simulink model "vdc_dyc_v3"  (R2020a)
settings: Solver=ode4  StartTime=0.0  StopTime=inf  FixedStep=1e-3  RelTol=1e-3
InitFcn:
  | clear mex
values from neighbouring files (symbols this model uses):
  vicrt_inputfile = append(path_send,              '2261_VOLCANO_ramp_RH12002_send_svm.xml')    [select_maneuver_files.m]
undefined symbols (not defined in the file or in its folder): vicrt_initcallback, vicrt_initmexcallback, vicrt_simulationmanager
libraries: simulink x1
(part 2 of 5)

== system vdc_dyc_v3/2261 VOLCANO PL7 MY22 R03/VI-CarRealTime/Input_Bus/Bus2Map ==
  Bus In : Inport
  Bus Selector : BusSelector  OutputSignals=Driver_Demands.str_swa,Subsystem_Activation.Internal_Steering_Column_Activity,Driver_Demands.rack_displacement,Driver_Demands.throttle,Driver_Demands.gear,Driver_Demands.clutch,Driver_Demands.brake,Driver_Demands.target_speed,Driver_Demands.target_acc,Brake_System_General.brk_mast_cyl_pres,Brake_System_General.brk_bias_front,ABS.Internal_ABS_Activity,ABS.ABS_threshold,Driver_Demands.user_maneuver_ID,Driver_Demands.user_input_steering,Driver_Demands.user_input_throttle,Driver_Demands.user_input_braking,Driver_Demands.user_input_gear,Driver_Demands.user_input_clutch,TCS.Internal_TCS_Activity,TCS.TCS_threshold,Friction.tire_mu.L1,Friction.tire_mu.L2,Friction.tire_mu.R1,Friction.tire_mu.R2,Subsystem_Activation.Internal_Brake_System_Activity.L1,Brake_System.brk_mmag_sign.L1,Brake_System.brk_mmag_unsign.L1,Brake_System.brk_pres.L1,Brake_System.brk_pres_gain.L1,Brake_System.brk_mu.L1,Subsystem_Activation.Internal_Brake_System_Activity.L2,Brake_System.brk_mmag_sign.L2,Brake_System.brk_mmag_unsign.L2,Brake_System.brk_pres.L2,Brake_System.brk_pres_gain.L2,Brake_System.brk_mu.L2,Subsystem_Activation.Internal_Brake_System_Activity.R1,Brake_System.brk_mmag_sign.R1,Brake_System.brk_mmag_unsign.R1,Brake_System.brk_pres.R1,Brake_System.brk_pres_gain.R1,Brake_System.brk_mu.R1,Subsystem_Activation.Internal_Brake_System_Activity.R2,Brake_System.brk_mmag_sign.R2,Brake_System.brk_mmag_unsign.R2,Brake_System.brk_pres.R2,Brake_System.brk_pres_gain.R2,Brake_System.brk_mu.R2,Hook.Fx.rear,Hook.Fy.rear,Hook.Fz.rear,Hook.Mx.rear,Hook.My.rear,Hook.Mz.rear,Rear_Steering_Actuator_disp.str_swa.left,Rear_Steering_Actuator_disp.str_swa.right,Steering.steer_at_spindle.L1,Steering.steer_at_spindle.L2,Steering.steer_at_spindle.R1,Steering.steer_at_spindle.R2,Steering.Internal_Hand_Wheel_Torque_Computation,Steering.Hand_Wheel_Torque,Subsystem_Activation.Internal_Clutch_Activity,Subsystem_Activation.Internal_Engine_Activity,Subsystem_Activation.Internal_Motor_to_Clutch_Activity,Subsystem_Activation.Internal_Motor_to_GearBox_Activity,Subsystem_Activation.Internal_Motor_to_CentralDifferential_Activity,Subsystem_Activation.Internal_Motor_to_FrontDifferential_Activity,Subsystem_Activation.Internal_Motor_to_RearDifferential_Activity,Subsystem_Activation.Internal_Motor_to_FrontRightWheel_Activity,Subsystem_Activation.Internal_Motor_to_FrontLeftWheel_Activity,Subsystem_Activation.Internal_Motor_to_RearRightWheel_Activity,Subsystem_Activation.Internal_Motor_to_RearLeftWheel_Activity,Subsystem_Activation.Internal_Engine_Idle_MaxRev_Controls_Activity,Subsystem_Activation.Internal_Gearbox_Activity,Subsystem_Activation.Internal_CentralDifferential_Activity,Subsystem_Activation.Internal_FrontDifferential_Activity,Subsystem_Activation.Internal_RearDifferential_Activity,Engine.engine_omega,Engine.engine_max_trq,Engine.engine_min_trq,Engine.engine_trq,Engine.clutch_inputplate_torque,Engine.non_termic_engine_trq,Engine.efficiency,Engine.throttle_scaling,Engine.control_mode,Engine.throttle_offset,GearBox.efficiency,GearBox.transmission_ratio,GearBox.diff_central_inputshaft_torque,GearBox.clutch_outputplate_angle,GearBox.clutch_outputplate_omega,GearBox.clutch_outputplate_alpha,GearBox.automatic_gearbox_shifting_mode,Clutch.clutch_trq,Clutch.gearbox_inputshaft_torque,Clutch.inputplate_angle,Clutch.inputplate_omega,Clutch.inputplate_alpha,Clutch.efficiency,Differential_Central.efficiency,Differential_Central.diff_front_inputshaft_torque,Differential_Central.diff_rear_inputshaft_torque,Differential_Central.gearbox_outputshaft_angle,Differential_Central.gearbox_outputshaft_omega,Differential_Central.gearbox_outputshaft_alpha,Differential_Front.efficiency,Differential_Front.wheel_front_left_torque,Differential_Front.wheel_front_right_torque,Differential_Front.diff_central_front_outputshaft_angle,Differential_Front.diff_central_front_outputshaft_omega,Differential_Front.diff_central_front_outputshaft_alpha,Differential_Rear.efficiency,Differential_Rear.wheel_rear_left_torque,Differential_Rear.wheel_rear_right_torque,Differential_Rear.diff_central_rear_outputshaft_angle,Differential_Rear.diff_central_rear_outputshaft_omega,Differential_Rear.diff_central_rear_outputshaft_alpha,Generic_Engine_to_Clutch.transmission_ratio,Generic_Engine_to_Clutch.regeneration_factor,Generic_Engine_to_Clutch.throttle_scaling,Generic_Engine_to_Clutch.control_mode,Generic_Engine_to_Clutch.throttle_offset,Generic_Engine_to_Clutch.efficiency,Generic_Engine_to_Clutch.engine_torque,Generic_Engine_to_Clutch.engine_max_torque,Generic_Engine_to_Clutch.engine_min_torque,Generic_Engine_to_Gearbox.transmission_ratio,Generic_Engine_to_Gearbox.regeneration_factor,Generic_Engine_to_Gearbox.throttle_scaling,Generic_Engine_to_Gearbox.control_mode,Generic_Engine_to_Gearbox.throttle_offset,Generic_Engine_to_Gearbox.efficiency,Generic_Engine_to_Gearbox.engine_torque,Generic_Engine_to_Gearbox.engine_max_torque,Generic_Engine_to_Gearbox.engine_min_torque,Generic_Engine_to_Central_Differential.transmission_ratio,Generic_Engine_to_Central_Differential.reverse_mode,Generic_Engine_to_Central_Differential.regeneration_factor,Generic_Engine_to_Central_Differential.throttle_scaling,Generic_Engine_to_Central_Differential.control_mode,Generic_Engine_to_Central_Differential.throttle_offset,Generic_Engine_to_Central_Differential.efficiency,Generic_Engine_to_Central_Differential.engine_torque,Generic_Engine_to_Central_Differential.engine_max_torque,Generic_Engine_to_Central_Differential.engine_min_torque,Generic_Engine_to_Front_Differential.transmission_ratio,Generic_Engine_to_Front_Differential.reverse_mode,Generic_Engine_to_Front_Differential.regeneration_factor,Generic_Engine_to_Front_Differential.throttle_scaling,Generic_Engine_to_Front_Differential.control_mode,Generic_Engine_to_Front_Differential.throttle_offset,Generic_Engine_to_Front_Differential.efficiency,Generic_Engine_to_Front_Differential.engine_torque,Generic_Engine_to_Front_Differential.engine_max_torque,Generic_Engine_to_Front_Differential.engine_min_torque,Generic_Engine_to_Rear_Differential.transmission_ratio,Generic_Engine_to_Rear_Differential.reverse_mode,Generic_Engine_to_Rear_Differential.regeneration_factor,Generic_Engine_to_Rear_Differential.throttle_scaling,Generic_Engine_to_Rear_Differential.control_mode,Generic_Engine_to_Rear_Differential.throttle_offset,Generic_Engine_to_Rear_Differential.efficiency,Generic_Engine_to_Rear_Differential.engine_torque,Generic_Engine_to_Rear_Differential.engine_max_torque,Generic_Engine_to_Rear_Differential.engine_min_torque,Generic_Engine_to_Front_Right_Wheel.transmission_ratio,Generic_Engine_to_Front_Right_Wheel.reverse_mode,Generic_Engine_to_Front_Right_Wheel.regeneration_factor,Generic_Engine_to_Front_Right_Wheel.throttle_scaling,Generic_Engine_to_Front_Right_Wheel.control_mode,Generic_Engine_to_Front_Right_Wheel.throttle_offset,Generic_Engine_to_Front_Right_Wheel.efficiency,Generic_Engine_to_Front_Right_Wheel.engine_torque,Generic_Engine_to_Front_Right_Wheel.engine_max_torque,Generic_Engine_to_Front_Right_Wheel.engine_min_torque,Generic_Engine_to_Front_Left_Wheel.transmission_ratio,Generic_Engine_to_Front_Left_Wheel.reverse_mode,Generic_Engine_to_Front_Left_Wheel.regeneration_factor,Generic_Engine_to_Front_Left_Wheel.throttle_scaling,Generic_Engine_to_Front_Left_Wheel.control_mode,Generic_Engine_to_Front_Left_Wheel.throttle_offset,Generic_Engine_to_Front_Left_Wheel.efficiency,Generic_Engine_to_Front_Left_Wheel.engine_torque,Generic_Engine_to_Front_Left_Wheel.engine_max_torque,Generic_Engine_to_Front_Left_Wheel.engine_min_torque,Generic_Engine_to_Rear_Right_Wheel.transmission_ratio,Generic_Engine_to_Rear_Right_Wheel.reverse_mode,Generic_Engine_to_Rear_Right_Wheel.regeneration_factor,Generic_Engine_to_Rear_Right_Wheel.throttle_scaling,Generic_Engine_to_Rear_Right_Wheel.control_mode,Generic_Engine_to_Rear_Right_Wheel.throttle_offset,Generic_Engine_to_Rear_Right_Wheel.efficiency,Generic_Engine_to_Rear_Right_Wheel.engine_torque,Generic_Engine_to_Rear_Right_Wheel.engine_max_torque,Generic_Engine_to_Rear_Right_Wheel.engine_min_torque,Generic_Engine_to_Rear_Left_Wheel.transmission_ratio,Generic_Engine_to_Rear_Left_Wheel.reverse_mode,Generic_Engine_to_Rear_Left_Wheel.regeneration_factor,Generic_Engine_to_Rear_Left_Wheel.throttle_scaling,Generic_Engine_to_Rear_Left_Wheel.control_mode,Generic_Engine_to_Rear_Left_Wheel.throttle_offset,Generic_Engine_to_Rear_Left_Wheel.efficiency,Generic_Engine_to_Rear_Left_Wheel.engine_torque,Generic_Engine_to_Rear_Left_Wheel.engine_max_torque,Generic_Engine_to_Rear_Left_Wheel.engine_min_torque,Antiroll_Bar.activity_flag.front,Antiroll_Bar.activity_flag.rear,Antiroll_Bar.force.front,Antiroll_Bar.force.rear,Subsystem_Activation.Internal_Aero_Activity,Aerodynamic.my_scaling,Aerodynamic.fx_central_scaling,Aerodynamic.fz_front_scaling,Aerodynamic.fz_rear_scaling,Aerodynamic.fx_front,Aerodynamic.fy_front,Aerodynamic.fz_front,Aerodynamic.fx_rear,Aerodynamic.fy_rear,Aerodynamic.fz_rear,Aerodynamic.fx_center,Aerodynamic.fy_center,Aerodynamic.fz_center,Aerodynamic.mx,Aerodynamic.my,Aerodynamic.mz,Irregularity.road.L1,Irregularity.road.L2,Irregularity.road.R1,Irregularity.road.R2,Main_Damper.force.L1,Main_Damper.activity_flag.L1,Main_Damper.force.L2,Main_Damper.activity_flag.L2,Main_Damper.force.R1,Main_Damper.activity_flag.R1,Main_Damper.force.R2,Main_Damper.activity_flag.R2,Main_Spring.force.L1,Main_Spring.activity_flag.L1,Main_Spring.force.L2,Main_Spring.activity_flag.L2,Main_Spring.force.R1,Main_Spring.activity_flag.R1,Main_Spring.force.R2,Main_Spring.activity_flag.R2,Main_Bumpstop.force.L1,Main_Bumpstop.activity_flag.L1,Main_Bumpstop.force.L2,Main_Bumpstop.activity_flag.L2,Main_Bumpstop.force.R1,Main_Bumpstop.activity_flag.R1,Main_Bumpstop.force.R2,Main_Bumpstop.activity_flag.R2,Main_Reboundstop.force.L1,Main_Reboundstop.activity_flag.L1,Main_Reboundstop.force.L2,Main_Reboundstop.activity_flag.L2,Main_Reboundstop.force.R1,Main_Reboundstop.activity_flag.R1,Main_Reboundstop.force.R2,Main_Reboundstop.activity_flag.R2,Auxiliary_vertical.force.L1,Auxiliary_vertical.activity_flag.L1,Auxiliary_vertical.force.L2,Auxiliary_vertical.activity_flag.L2,Auxiliary_vertical.force.R1,Auxiliary_vertical.activity_flag.R1,Auxiliary_vertical.force.R2,Auxiliary_vertical.activity_flag.R2,Main_Inerter.force.L1,Main_Inerter.activity_flag.L1,Main_Inerter.force.L2,Main_Inerter.activity_flag.L2,Main_Inerter.force.R1,Main_Inerter.activity_flag.R1,Main_Inerter.force.R2,Main_Inerter.activity_flag.R2,Third_Element.Damper_force.front,Third_Element.Damper_activity_flag.front,Third_Element.Damper_force.rear,Third_Element.Damper_activity_flag.rear,Third_Element.Spring.front,Third_Element.Spring_activity_flag.front,Third_Element.Spring.rear,Third_Element.Spring_activity_flag.rear,Mono_Element.Damper.front,Mono_Element.Damper_activity_flag.front,Mono_Element.Damper.rear,Mono_Element.Damper_activity_flag.rear,Mono_Element.Inerter.front,Mono_Element.Inerter_activity_flag.front,Mono_Element.Inerter.rear,Mono_Element.Inerter_activity_flag.rear,Mono_Element.Spring.front,Mono_Element.Spring_activity_flag.front,Mono_Element.Spring.rear,Mono_Element.Spring_activity_flag.rear,Mono_Element.Bumpstop_Spring.front,Mono_Element.Bumpstop_Spring_activity_flag.front,Mono_Element.Bumpstop_Spring.rear,Mono_Element.Bumpstop_Spring_activity_flag.rear,Mono_Element.Reboundstop_Spring.front,Mono_Element.Reboundstop_Spring_activity_flag.front,Mono_Element.Reboundstop_Spring.rear,Mono_Element.Reboundstop_Spring_activity_flag.rear,Mono_Element.Bumpstop_Damper.front,Mono_Element.Bumpstop_Damper_activity_flag.front,Mono_Element.Bumpstop_Damper.rear,Mono_Element.Bumpstop_Damper_activity_flag.rear,Mono_Element.Reboundstop_Damper.front,Mono_Element.Reboundstop_Damper_activity_flag.front,Mono_Element.Reboundstop_Damper.rear,Mono_Element.Reboundstop_Damper_activity_flag.rear,Mono_Element.Roll_Damper.front,Mono_Element.Roll_Damper_activity_flag.front,Mono_Element.Roll_Damper.rear,Mono_Element.Roll_Damper_activity_flag.rear,Subsystem_Activation.Tire_Force_x.L1,Subsystem_Activation.Tire_Force_y.L1,Subsystem_Activation.Tire_Force_z.L1,Subsystem_Activation.Tire_Moment_x.L1,Subsystem_Activation.Tire_Moment_y.L1,Subsystem_Activation.Tire_Moment_z.L1,Tire_Force.Fx.L1,Tire_Force.Fy.L1,Tire_Force.Fz.L1,Tire_Moment.Mx.L1,Tire_Moment.My.L1,Tire_Moment.Mz.L1,Subsystem_Activation.Tire_Force_x.L2,Subsystem_Activation.Tire_Force_y.L2,Subsystem_Activation.Tire_Force_z.L2,Subsystem_Activation.Tire_Moment_x.L2,Subsystem_Activation.Tire_Moment_y.L2,Subsystem_Activation.Tire_Moment_z.L2,Tire_Force.Fx.L2,Tire_Force.Fy.L2,Tire_Force.Fz.L2,Tire_Moment.Mx.L2,Tire_Moment.My.L2,Tire_Moment.Mz.L2,Subsystem_Activation.Tire_Force_x.R1,Subsystem_Activation.Tire_Force_y.R1,Subsystem_Activation.Tire_Force_z.R1,Subsystem_Activation.Tire_Moment_x.R1,Subsystem_Activation.Tire_Moment_y.R1,Subsystem_Activation.Tire_Moment_z.R1,Tire_Force.Fx.R1,Tire_Force.Fy.R1,Tire_Force.Fz.R1,Tire_Moment.Mx.R1,Tire_Moment.My.R1,Tire_Moment.Mz.R1,Subsystem_Activation.Tire_Force_x.R2,Subsystem_Activation.Tire_Force_y.R2,Subsystem_Activation.Tire_Force_z.R2,Subsystem_Activation.Tire_Moment_x.R2,Subsystem_Activation.Tire_Moment_y.R2,Subsystem_Activation.Tire_Moment_z.R2,Tire_Force.Fx.R2,Tire_Force.Fy.R2,Tire_Force.Fz.R2,Tire_Moment.Mx.R2,Tire_Moment.My.R2,Tire_Moment.Mz.R2,Wheel_driving.moment.L1,Wheel_driving.moment.L2,Wheel_driving.moment.R1,Wheel_driving.moment.R2,Ext_Body.force.X,Ext_Body.force.Y,Ext_Body.force.Z,Ext_Body.moment.X,Ext_Body.moment.Y,Ext_Body.moment.Z,Ext_Ground.force.X,Ext_Ground.force.Y,Ext_Ground.force.Z,Ext_Ground.moment.X,Ext_Ground.moment.Y,Ext_Ground.moment.Z,Ext_Tracking.force.X,Ext_Tracking.force.Y,Ext_Tracking.moment.X,Ext_Tracking.moment.Y
  Mux : Mux  Inputs=389
  Map Out : Outport  VectorParamsAs1DForOutWhenUnconnected=off
  wires:
  Mux/1 -> Map Out/1
  Bus In/1 -> Bus Selector/1
  Bus Selector/1 -> Mux/1  "<str_swa>"
  Bus Selector/2 -> Mux/2  "<Internal_Steering_Column_Activity>"
  Bus Selector/3 -> Mux/3  "<rack_displacement>"
  Bus Selector/4 -> Mux/4  "<throttle>"
  Bus Selector/5 -> Mux/5  "<gear>"
  Bus Selector/6 -> Mux/6  "<clutch>"
  Bus Selector/7 -> Mux/7  "<brake>"
  Bus Selector/8 -> Mux/8  "<target_speed>"
  Bus Selector/9 -> Mux/9  "<target_acc>"
  Bus Selector/10 -> Mux/10  "<brk_mast_cyl_pres>"
  Bus Selector/11 -> Mux/11  "<brk_bias_front>"
  Bus Selector/12 -> Mux/12  "<Internal_ABS_Activity>"
  Bus Selector/13 -> Mux/13  "<ABS_threshold>"
  Bus Selector/14 -> Mux/14  "<user_maneuver_ID>"
  Bus Selector/15 -> Mux/15  "<user_input_steering>"
  Bus Selector/16 -> Mux/16  "<user_input_throttle>"
  Bus Selector/17 -> Mux/17  "<user_input_braking>"
  Bus Selector/18 -> Mux/18  "<user_input_gear>"
  Bus Selector/19 -> Mux/19  "<user_input_clutch>"
  Bus Selector/20 -> Mux/20  "<Internal_TCS_Activity>"
  Bus Selector/21 -> Mux/21  "<TCS_threshold>"
  Bus Selector/22 -> Mux/22  "<L1>"
  Bus Selector/23 -> Mux/23  "<L2>"
  Bus Selector/24 -> Mux/24  "<R1>"
  Bus Selector/25 -> Mux/25  "<R2>"
  Bus Selector/26 -> Mux/26  "<L1>"
  Bus Selector/27 -> Mux/27  "<L1>"
  Bus Selector/28 -> Mux/28  "<L1>"
  Bus Selector/29 -> Mux/29  "<L1>"
  Bus Selector/30 -> Mux/30  "<L1>"
  Bus Selector/31 -> Mux/31  "<L1>"
  Bus Selector/32 -> Mux/32  "<L2>"
  Bus Selector/33 -> Mux/33  "<L2>"
  Bus Selector/34 -> Mux/34  "<L2>"
  Bus Selector/35 -> Mux/35  "<L2>"
  Bus Selector/36 -> Mux/36  "<L2>"
  Bus Selector/37 -> Mux/37  "<L2>"
  Bus Selector/38 -> Mux/38  "<R1>"
  Bus Selector/39 -> Mux/39  "<R1>"
  Bus Selector/40 -> Mux/40  "<R1>"
  Bus Selector/41 -> Mux/41  "<R1>"
  Bus Selector/42 -> Mux/42  "<R1>"
  Bus Selector/43 -> Mux/43  "<R1>"
  Bus Selector/44 -> Mux/44  "<R2>"
  Bus Selector/45 -> Mux/45  "<R2>"
  Bus Selector/46 -> Mux/46  "<R2>"
  Bus Selector/47 -> Mux/47  "<R2>"
  Bus Selector/48 -> Mux/48  "<R2>"
  Bus Selector/49 -> Mux/49  "<R2>"
  Bus Selector/50 -> Mux/50  "<rear>"
  Bus Selector/51 -> Mux/51  "<rear>"
  Bus Selector/52 -> Mux/52  "<rear>"
  Bus Selector/53 -> Mux/53  "<rear>"
  Bus Selector/54 -> Mux/54  "<rear>"
  Bus Selector/55 -> Mux/55  "<rear>"
  Bus Selector/56 -> Mux/56  "<left>"
  Bus Selector/57 -> Mux/57  "<right>"
  Bus Selector/58 -> Mux/58  "<L1>"
  Bus Selector/59 -> Mux/59  "<L2>"
  Bus Selector/60 -> Mux/60  "<R1>"
  Bus Selector/61 -> Mux/61  "<R2>"
  Bus Selector/62 -> Mux/62  "<Internal_Hand_Wheel_Torque_Computation>"
  Bus Selector/63 -> Mux/63  "<Hand_Wheel_Torque>"
  Bus Selector/64 -> Mux/64  "<Internal_Clutch_Activity>"
  Bus Selector/65 -> Mux/65  "<Internal_Engine_Activity>"
  Bus Selector/66 -> Mux/66  "<Internal_Motor_to_Clutch_Activity>"
  Bus Selector/67 -> Mux/67  "<Internal_Motor_to_GearBox_Activity>"
  Bus Selector/68 -> Mux/68  "<Internal_Motor_to_CentralDifferential_Activity>"
  Bus Selector/69 -> Mux/69  "<Internal_Motor_to_FrontDifferential_Activity>"
  Bus Selector/70 -> Mux/70  "<Internal_Motor_to_RearDifferential_Activity>"
  Bus Selector/71 -> Mux/71  "<Internal_Motor_to_FrontRightWheel_Activity>"
  Bus Selector/72 -> Mux/72  "<Internal_Motor_to_FrontLeftWheel_Activity>"
  Bus Selector/73 -> Mux/73  "<Internal_Motor_to_RearRightWheel_Activity>"
  Bus Selector/74 -> Mux/74  "<Internal_Motor_to_RearLeftWheel_Activity>"
  Bus Selector/75 -> Mux/75  "<Internal_Engine_Idle_MaxRev_Controls_Activity>"
  Bus Selector/76 -> Mux/76  "<Internal_Gearbox_Activity>"
  Bus Selector/77 -> Mux/77  "<Internal_CentralDifferential_Activity>"
  Bus Selector/78 -> Mux/78  "<Internal_FrontDifferential_Activity>"
  Bus Selector/79 -> Mux/79  "<Internal_RearDifferential_Activity>"
  Bus Selector/80 -> Mux/80  "<engine_omega>"
  Bus Selector/81 -> Mux/81  "<engine_max_trq>"
  Bus Selector/82 -> Mux/82  "<engine_min_trq>"
  Bus Selector/83 -> Mux/83  "<engine_trq>"
  Bus Selector/84 -> Mux/84  "<clutch_inputplate_torque>"
  Bus Selector/85 -> Mux/85  "<non_termic_engine_trq>"
  Bus Selector/86 -> Mux/86  "<efficiency>"
  Bus Selector/87 -> Mux/87  "<throttle_scaling>"
  Bus Selector/88 -> Mux/88  "<control_mode>"
  Bus Selector/89 -> Mux/89  "<throttle_offset>"
  Bus Selector/90 -> Mux/90  "<efficiency>"
  Bus Selector/91 -> Mux/91  "<transmission_ratio>"
  Bus Selector/92 -> Mux/92  "<diff_central_inputshaft_torque>"
  Bus Selector/93 -> Mux/93  "<clutch_outputplate_angle>"
  Bus Selector/94 -> Mux/94  "<clutch_outputplate_omega>"
  Bus Selector/95 -> Mux/95  "<clutch_outputplate_alpha>"
  Bus Selector/96 -> Mux/96  "<automatic_gearbox_shifting_mode>"
  Bus Selector/97 -> Mux/97  "<clutch_trq>"
  Bus Selector/98 -> Mux/98  "<gearbox_inputshaft_torque>"
  Bus Selector/99 -> Mux/99  "<inputplate_angle>"
  Bus Selector/100 -> Mux/100  "<inputplate_omega>"
  Bus Selector/101 -> Mux/101  "<inputplate_alpha>"
  Bus Selector/102 -> Mux/102  "<efficiency>"
  Bus Selector/103 -> Mux/103  "<efficiency>"
  Bus Selector/104 -> Mux/104  "<diff_front_inputshaft_torque>"
  Bus Selector/105 -> Mux/105  "<diff_rear_inputshaft_torque>"
  Bus Selector/106 -> Mux/106  "<gearbox_outputshaft_angle>"
  Bus Selector/107 -> Mux/107  "<gearbox_outputshaft_omega>"
  Bus Selector/108 -> Mux/108  "<gearbox_outputshaft_alpha>"
  Bus Selector/109 -> Mux/109  "<efficiency>"
  Bus Selector/110 -> Mux/110  "<wheel_front_left_torque>"
  Bus Selector/111 -> Mux/111  "<wheel_front_right_torque>"
  Bus Selector/112 -> Mux/112  "<diff_central_front_outputshaft_angle>"
  Bus Selector/113 -> Mux/113  "<diff_central_front_outputshaft_omega>"
  Bus Selector/114 -> Mux/114  "<diff_central_front_outputshaft_alpha>"
  Bus Selector/115 -> Mux/115  "<efficiency>"
  Bus Selector/116 -> Mux/116  "<wheel_rear_left_torque>"
  Bus Selector/117 -> Mux/117  "<wheel_rear_right_torque>"
  Bus Selector/118 -> Mux/118  "<diff_central_rear_outputshaft_angle>"
  Bus Selector/119 -> Mux/119  "<diff_central_rear_outputshaft_omega>"
  Bus Selector/120 -> Mux/120  "<diff_central_rear_outputshaft_alpha>"
  Bus Selector/121 -> Mux/121  "<transmission_ratio>"
  Bus Selector/122 -> Mux/122  "<regeneration_factor>"
  Bus Selector/123 -> Mux/123  "<throttle_scaling>"
  Bus Selector/124 -> Mux/124  "<control_mode>"
  Bus Selector/125 -> Mux/125  "<throttle_offset>"
  Bus Selector/126 -> Mux/126  "<efficiency>"
  Bus Selector/127 -> Mux/127  "<engine_torque>"
  Bus Selector/128 -> Mux/128  "<engine_max_torque>"
  Bus Selector/129 -> Mux/129  "<engine_min_torque>"
  Bus Selector/130 -> Mux/130  "<transmission_ratio>"
  Bus Selector/131 -> Mux/131  "<regeneration_factor>"
  Bus Selector/132 -> Mux/132  "<throttle_scaling>"
  Bus Selector/133 -> Mux/133  "<control_mode>"
  Bus Selector/134 -> Mux/134  "<throttle_offset>"
  Bus Selector/135 -> Mux/135  "<efficiency>"
  Bus Selector/136 -> Mux/136  "<engine_torque>"
  Bus Selector/137 -> Mux/137  "<engine_max_torque>"
  Bus Selector/138 -> Mux/138  "<engine_min_torque>"
  Bus Selector/139 -> Mux/139  "<transmission_ratio>"
  Bus Selector/140 -> Mux/140  "<reverse_mode>"
  Bus Selector/141 -> Mux/141  "<regeneration_factor>"
  Bus Selector/142 -> Mux/142  "<throttle_scaling>"
  Bus Selector/143 -> Mux/143  "<control_mode>"
  Bus Selector/144 -> Mux/144  "<throttle_offset>"
  Bus Selector/145 -> Mux/145  "<efficiency>"
  Bus Selector/146 -> Mux/146  "<engine_torque>"
  Bus Selector/147 -> Mux/147  "<engine_max_torque>"
  Bus Selector/148 -> Mux/148  "<engine_min_torque>"
  Bus Selector/149 -> Mux/149  "<transmission_ratio>"
  Bus Selector/150 -> Mux/150  "<reverse_mode>"
  Bus Selector/151 -> Mux/151  "<regeneration_factor>"
  Bus Selector/152 -> Mux/152  "<throttle_scaling>"
  Bus Selector/153 -> Mux/153  "<control_mode>"
  Bus Selector/154 -> Mux/154  "<throttle_offset>"
  Bus Selector/155 -> Mux/155  "<efficiency>"
  Bus Selector/156 -> Mux/156  "<engine_torque>"
  Bus Selector/157 -> Mux/157  "<engine_max_torque>"
  Bus Selector/158 -> Mux/158  "<engine_min_torque>"
  Bus Selector/159 -> Mux/159  "<transmission_ratio>"
  Bus Selector/160 -> Mux/160  "<reverse_mode>"
  Bus Selector/161 -> Mux/161  "<regeneration_factor>"
  Bus Selector/162 -> Mux/162  "<throttle_scaling>"
  Bus Selector/163 -> Mux/163  "<control_mode>"
  Bus Selector/164 -> Mux/164  "<throttle_offset>"
  Bus Selector/165 -> Mux/165  "<efficiency>"
  Bus Selector/166 -> Mux/166  "<engine_torque>"
  Bus Selector/167 -> Mux/167  "<engine_max_torque>"
  Bus Selector/168 -> Mux/168  "<engine_min_torque>"
  Bus Selector/169 -> Mux/169  "<transmission_ratio>"
  Bus Selector/170 -> Mux/170  "<reverse_mode>"
  Bus Selector/171 -> Mux/171  "<regeneration_factor>"
  Bus Selector/172 -> Mux/172  "<throttle_scaling>"
  Bus Selector/173 -> Mux/173  "<control_mode>"
  Bus Selector/174 -> Mux/174  "<throttle_offset>"
  Bus Selector/175 -> Mux/175  "<efficiency>"
  Bus Selector/176 -> Mux/176  "<engine_torque>"
  Bus Selector/177 -> Mux/177  "<engine_max_torque>"
  Bus Selector/178 -> Mux/178  "<engine_min_torque>"
  Bus Selector/179 -> Mux/179  "<transmission_ratio>"
  Bus Selector/180 -> Mux/180  "<reverse_mode>"
  Bus Selector/181 -> Mux/181  "<regeneration_factor>"
  Bus Selector/182 -> Mux/182  "<throttle_scaling>"
  Bus Selector/183 -> Mux/183  "<control_mode>"
  Bus Selector/184 -> Mux/184  "<throttle_offset>"
  Bus Selector/185 -> Mux/185  "<efficiency>"
  Bus Selector/186 -> Mux/186  "<engine_torque>"
  Bus Selector/187 -> Mux/187  "<engine_max_torque>"
  Bus Selector/188 -> Mux/188  "<engine_min_torque>"
  Bus Selector/189 -> Mux/189  "<transmission_ratio>"
  Bus Selector/190 -> Mux/190  "<reverse_mode>"
  Bus Selector/191 -> Mux/191  "<regeneration_factor>"
  Bus Selector/192 -> Mux/192  "<throttle_scaling>"
  Bus Selector/193 -> Mux/193  "<control_mode>"
  Bus Selector/194 -> Mux/194  "<throttle_offset>"
  Bus Selector/195 -> Mux/195  "<efficiency>"
  Bus Selector/196 -> Mux/196  "<engine_torque>"
  Bus Selector/197 -> Mux/197  "<engine_max_torque>"
  Bus Selector/198 -> Mux/198  "<engine_min_torque>"
  Bus Selector/199 -> Mux/199  "<transmission_ratio>"
  Bus Selector/200 -> Mux/200  "<reverse_mode>"
  Bus Selector/201 -> Mux/201  "<regeneration_factor>"
  Bus Selector/202 -> Mux/202  "<throttle_scaling>"
  Bus Selector/203 -> Mux/203  "<control_mode>"
  Bus Selector/204 -> Mux/204  "<throttle_offset>"
  Bus Selector/205 -> Mux/205  "<efficiency>"
  Bus Selector/206 -> Mux/206  "<engine_torque>"
  Bus Selector/207 -> Mux/207  "<engine_max_torque>"
  Bus Selector/208 -> Mux/208  "<engine_min_torque>"
  Bus Selector/209 -> Mux/209  "<front>"
  Bus Selector/210 -> Mux/210  "<rear>"
  Bus Selector/211 -> Mux/211  "<front>"
  Bus Selector/212 -> Mux/212  "<rear>"
  Bus Selector/213 -> Mux/213  "<Internal_Aero_Activity>"
  Bus Selector/214 -> Mux/214  "<my_scaling>"
  Bus Selector/215 -> Mux/215  "<fx_central_scaling>"
  Bus Selector/216 -> Mux/216  "<fz_front_scaling>"
  Bus Selector/217 -> Mux/217  "<fz_rear_scaling>"
  Bus Selector/218 -> Mux/218  "<fx_front>"
  Bus Selector/219 -> Mux/219  "<fy_front>"
  Bus Selector/220 -> Mux/220  "<fz_front>"
  Bus Selector/221 -> Mux/221  "<fx_rear>"
  Bus Selector/222 -> Mux/222  "<fy_rear>"
  Bus Selector/223 -> Mux/223  "<fz_rear>"
  Bus Selector/224 -> Mux/224  "<fx_center>"
  Bus Selector/225 -> Mux/225  "<fy_center>"
  Bus Selector/226 -> Mux/226  "<fz_center>"
  Bus Selector/227 -> Mux/227  "<mx>"
  Bus Selector/228 -> Mux/228  "<my>"
  Bus Selector/229 -> Mux/229  "<mz>"
  Bus Selector/230 -> Mux/230  "<L1>"
  Bus Selector/231 -> Mux/231  "<L2>"
  Bus Selector/232 -> Mux/232  "<R1>"
  Bus Selector/233 -> Mux/233  "<R2>"
  Bus Selector/234 -> Mux/234  "<L1>"
  Bus Selector/235 -> Mux/235  "<L1>"
  Bus Selector/236 -> Mux/236  "<L2>"
  Bus Selector/237 -> Mux/237  "<L2>"
  Bus Selector/238 -> Mux/238  "<R1>"
  Bus Selector/239 -> Mux/239  "<R1>"
  Bus Selector/240 -> Mux/240  "<R2>"
  Bus Selector/241 -> Mux/241  "<R2>"
  Bus Selector/242 -> Mux/242  "<L1>"
  Bus Selector/243 -> Mux/243  "<L1>"
  Bus Selector/244 -> Mux/244  "<L2>"
  Bus Selector/245 -> Mux/245  "<L2>"
  Bus Selector/246 -> Mux/246  "<R1>"
  Bus Selector/247 -> Mux/247  "<R1>"
  Bus Selector/248 -> Mux/248  "<R2>"
  Bus Selector/249 -> Mux/249  "<R2>"
  Bus Selector/250 -> Mux/250  "<L1>"
  Bus Selector/251 -> Mux/251  "<L1>"
  Bus Selector/252 -> Mux/252  "<L2>"
  Bus Selector/253 -> Mux/253  "<L2>"
  Bus Selector/254 -> Mux/254  "<R1>"
  Bus Selector/255 -> Mux/255  "<R1>"
  Bus Selector/256 -> Mux/256  "<R2>"
  Bus Selector/257 -> Mux/257  "<R2>"
  Bus Selector/258 -> Mux/258  "<L1>"
  Bus Selector/259 -> Mux/259  "<L1>"
  Bus Selector/260 -> Mux/260  "<L2>"
  Bus Selector/261 -> Mux/261  "<L2>"
  Bus Selector/262 -> Mux/262  "<R1>"
  Bus Selector/263 -> Mux/263  "<R1>"
  Bus Selector/264 -> Mux/264  "<R2>"
  Bus Selector/265 -> Mux/265  "<R2>"
  Bus Selector/266 -> Mux/266  "<L1>"
  Bus Selector/267 -> Mux/267  "<L1>"
  Bus Selector/268 -> Mux/268  "<L2>"
  Bus Selector/269 -> Mux/269  "<L2>"
  Bus Selector/270 -> Mux/270  "<R1>"
  Bus Selector/271 -> Mux/271  "<R1>"
  Bus Selector/272 -> Mux/272  "<R2>"
  Bus Selector/273 -> Mux/273  "<R2>"
  Bus Selector/274 -> Mux/274  "<L1>"
  Bus Selector/275 -> Mux/275  "<L1>"
  Bus Selector/276 -> Mux/276  "<L2>"
  Bus Selector/277 -> Mux/277  "<L2>"
  Bus Selector/278 -> Mux/278  "<R1>"
  Bus Selector/279 -> Mux/279  "<R1>"
  Bus Selector/280 -> Mux/280  "<R2>"
  Bus Selector/281 -> Mux/281  "<R2>"
  Bus Selector/282 -> Mux/282  "<front>"
  Bus Selector/283 -> Mux/283  "<front>"
  Bus Selector/284 -> Mux/284  "<rear>"
  Bus Selector/285 -> Mux/285  "<rear>"
  Bus Selector/286 -> Mux/286  "<front>"
  Bus Selector/287 -> Mux/287  "<front>"
  Bus Selector/288 -> Mux/288  "<rear>"
  Bus Selector/289 -> Mux/289  "<rear>"
  Bus Selector/290 -> Mux/290  "<front>"
  Bus Selector/291 -> Mux/291  "<front>"
  Bus Selector/292 -> Mux/292  "<rear>"
  Bus Selector/293 -> Mux/293  "<rear>"
  Bus Selector/294 -> Mux/294  "<front>"
  Bus Selector/295 -> Mux/295  "<front>"
  Bus Selector/296 -> Mux/296  "<rear>"
  Bus Selector/297 -> Mux/297  "<rear>"
  Bus Selector/298 -> Mux/298  "<front>"
  Bus Selector/299 -> Mux/299  "<front>"
  Bus Selector/300 -> Mux/300  "<rear>"
  Bus Selector/301 -> Mux/301  "<rear>"
  Bus Selector/302 -> Mux/302  "<front>"
  Bus Selector/303 -> Mux/303  "<front>"
  Bus Selector/304 -> Mux/304  "<rear>"
  Bus Selector/305 -> Mux/305  "<rear>"
  Bus Selector/306 -> Mux/306  "<front>"
  Bus Selector/307 -> Mux/307  "<front>"
  Bus Selector/308 -> Mux/308  "<rear>"
  Bus Selector/309 -> Mux/309  "<rear>"
  Bus Selector/310 -> Mux/310  "<front>"
  Bus Selector/311 -> Mux/311  "<front>"
  Bus Selector/312 -> Mux/312  "<rear>"
  Bus Selector/313 -> Mux/313  "<rear>"
  Bus Selector/314 -> Mux/314  "<front>"
  Bus Selector/315 -> Mux/315  "<front>"
  Bus Selector/316 -> Mux/316  "<rear>"
  Bus Selector/317 -> Mux/317  "<rear>"
  Bus Selector/318 -> Mux/318  "<front>"
  Bus Selector/319 -> Mux/319  "<front>"
  Bus Selector/320 -> Mux/320  "<rear>"
  Bus Selector/321 -> Mux/321  "<rear>"
  Bus Selector/322 -> Mux/322  "<L1>"
  Bus Selector/323 -> Mux/323  "<L1>"
  Bus Selector/324 -> Mux/324  "<L1>"
  Bus Selector/325 -> Mux/325  "<L1>"
  Bus Selector/326 -> Mux/326  "<L1>"
  Bus Selector/327 -> Mux/327  "<L1>"
  Bus Selector/328 -> Mux/328  "<L1>"
  Bus Selector/329 -> Mux/329  "<L1>"
  Bus Selector/330 -> Mux/330  "<L1>"
  Bus Selector/331 -> Mux/331  "<L1>"
  Bus Selector/332 -> Mux/332  "<L1>"
  Bus Selector/333 -> Mux/333  "<L1>"
  Bus Selector/334 -> Mux/334  "<L2>"
  Bus Selector/335 -> Mux/335  "<L2>"
  Bus Selector/336 -> Mux/336  "<L2>"
  Bus Selector/337 -> Mux/337  "<L2>"
  Bus Selector/338 -> Mux/338  "<L2>"
  Bus Selector/339 -> Mux/339  "<L2>"
  Bus Selector/340 -> Mux/340  "<L2>"
  Bus Selector/341 -> Mux/341  "<L2>"
  Bus Selector/342 -> Mux/342  "<L2>"
  Bus Selector/343 -> Mux/343  "<L2>"
  Bus Selector/344 -> Mux/344  "<L2>"
  Bus Selector/345 -> Mux/345  "<L2>"
  Bus Selector/346 -> Mux/346  "<R1>"
  Bus Selector/347 -> Mux/347  "<R1>"
  Bus Selector/348 -> Mux/348  "<R1>"
  Bus Selector/349 -> Mux/349  "<R1>"
  Bus Selector/350 -> Mux/350  "<R1>"
  Bus Selector/351 -> Mux/351  "<R1>"
  Bus Selector/352 -> Mux/352  "<R1>"
  Bus Selector/353 -> Mux/353  "<R1>"
  Bus Selector/354 -> Mux/354  "<R1>"
  Bus Selector/355 -> Mux/355  "<R1>"
  Bus Selector/356 -> Mux/356  "<R1>"
  Bus Selector/357 -> Mux/357  "<R1>"
  Bus Selector/358 -> Mux/358  "<R2>"
  Bus Selector/359 -> Mux/359  "<R2>"
  Bus Selector/360 -> Mux/360  "<R2>"
  Bus Selector/361 -> Mux/361  "<R2>"
  Bus Selector/362 -> Mux/362  "<R2>"
  Bus Selector/363 -> Mux/363  "<R2>"
  Bus Selector/364 -> Mux/364  "<R2>"
  Bus Selector/365 -> Mux/365  "<R2>"
  Bus Selector/366 -> Mux/366  "<R2>"
  Bus Selector/367 -> Mux/367  "<R2>"
  Bus Selector/368 -> Mux/368  "<R2>"
  Bus Selector/369 -> Mux/369  "<R2>"
  Bus Selector/370 -> Mux/370  "<L1>"
  Bus Selector/371 -> Mux/371  "<L2>"
  Bus Selector/372 -> Mux/372  "<R1>"
  Bus Selector/373 -> Mux/373  "<R2>"
  Bus Selector/374 -> Mux/374  "<X>"
  Bus Selector/375 -> Mux/375  "<Y>"
  Bus Selector/376 -> Mux/376  "<Z>"
  Bus Selector/377 -> Mux/377  "<X>"
  Bus Selector/378 -> Mux/378  "<Y>"
  Bus Selector/379 -> Mux/379  "<Z>"
  Bus Selector/380 -> Mux/380  "<X>"
  Bus Selector/381 -> Mux/381  "<Y>"
  Bus Selector/382 -> Mux/382  "<Z>"
  Bus Selector/383 -> Mux/383  "<X>"
  Bus Selector/384 -> Mux/384  "<Y>"
  Bus Selector/385 -> Mux/385  "<Z>"
  Bus Selector/386 -> Mux/386  "<X>"
  Bus Selector/387 -> Mux/387  "<Y>"
  Bus Selector/388 -> Mux/388  "<X>"
  Bus Selector/389 -> Mux/389  "<Y>"

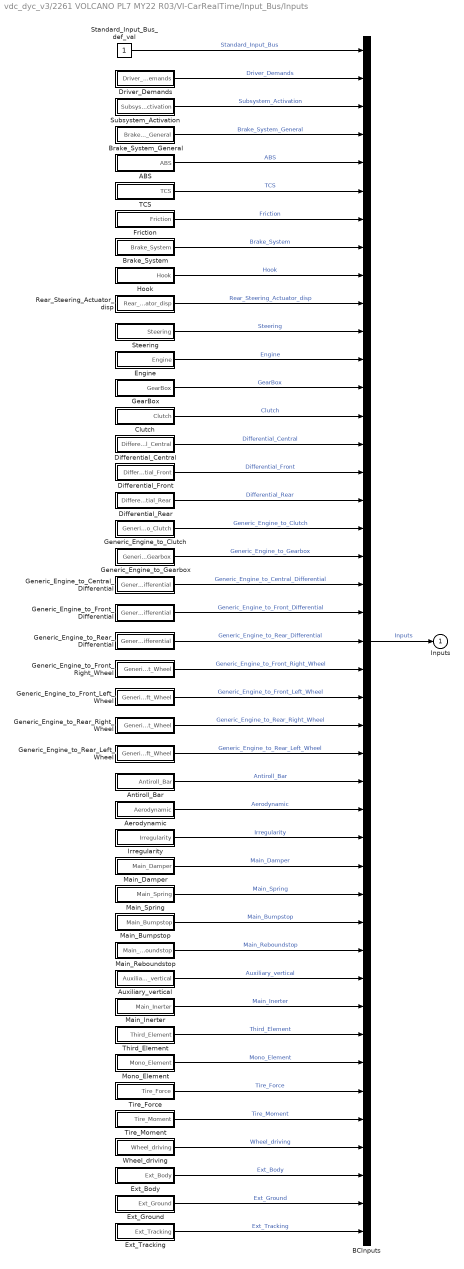
== system vdc_dyc_v3/2261 VOLCANO PL7 MY22 R03/VI-CarRealTime/Input_Bus/Inputs ==
  ABS : Subsystem
  Aerodynamic : Subsystem
  Antiroll_Bar : Subsystem
  Auxiliary_vertical : Subsystem
  BCInputs : BusCreator  Inputs=43
  Brake_System : Subsystem
  Brake_System_General : Subsystem
  Clutch : Subsystem
  Differential_Central : Subsystem
  Differential_Front : Subsystem
  Differential_Rear : Subsystem
  Driver_Demands : Subsystem
  Engine : Subsystem
  Ext_Body : Subsystem
  Ext_Ground : Subsystem
  Ext_Tracking : Subsystem
  Friction : Subsystem
  GearBox : Subsystem
  Generic_Engine_to_Central_Differential : Subsystem
  Generic_Engine_to_Clutch : Subsystem
  Generic_Engine_to_Front_Differential : Subsystem
  Generic_Engine_to_Front_Left_Wheel : Subsystem
  Generic_Engine_to_Front_Right_Wheel : Subsystem
  Generic_Engine_to_Gearbox : Subsystem
  Generic_Engine_to_Rear_Differential : Subsystem
  Generic_Engine_to_Rear_Left_Wheel : Subsystem
  Generic_Engine_to_Rear_Right_Wheel : Subsystem
  Hook : Subsystem
  Irregularity : Subsystem
  Main_Bumpstop : Subsystem
  Main_Damper : Subsystem
  Main_Inerter : Subsystem
  Main_Reboundstop : Subsystem
  Main_Spring : Subsystem
  Mono_Element : Subsystem
  Rear_Steering_Actuator_disp : Subsystem
  Standard_Input_Bus_def_val : Constant
  Steering : Subsystem
  Subsystem_Activation : Subsystem
  TCS : Subsystem
  Third_Element : Subsystem
  Tire_Force : Subsystem
  Tire_Moment : Subsystem
  Wheel_driving : Subsystem
  Inputs : Outport
  wires:
  BCInputs/1 -> Inputs/1  "Inputs"
  Standard_Input_Bus_def_val/1 -> BCInputs/1  "Standard_Input_Bus"
  Driver_Demands/1(Driver_Demands) -> BCInputs/2  "Driver_Demands"
  Subsystem_Activation/1(Subsystem_Activation) -> BCInputs/3  "Subsystem_Activation"
  Brake_System_General/1(Brake_System_General) -> BCInputs/4  "Brake_System_General"
  ABS/1(ABS) -> BCInputs/5  "ABS"
  TCS/1(TCS) -> BCInputs/6  "TCS"
  Friction/1(Friction) -> BCInputs/7  "Friction"
  Brake_System/1(Brake_System) -> BCInputs/8  "Brake_System"
  Hook/1(Hook) -> BCInputs/9  "Hook"
  Rear_Steering_Actuator_disp/1(Rear_Steering_Actuator_disp) -> BCInputs/10  "Rear_Steering_Actuator_disp"
  Steering/1(Steering) -> BCInputs/11  "Steering"
  Engine/1(Engine) -> BCInputs/12  "Engine"
  GearBox/1(GearBox) -> BCInputs/13  "GearBox"
  Clutch/1(Clutch) -> BCInputs/14  "Clutch"
  Differential_Central/1(Differential_Central) -> BCInputs/15  "Differential_Central"
  Differential_Front/1(Differential_Front) -> BCInputs/16  "Differential_Front"
  Differential_Rear/1(Differential_Rear) -> BCInputs/17  "Differential_Rear"
  Generic_Engine_to_Clutch/1(Generic_Engine_to_Clutch) -> BCInputs/18  "Generic_Engine_to_Clutch"
  Generic_Engine_to_Gearbox/1(Generic_Engine_to_Gearbox) -> BCInputs/19  "Generic_Engine_to_Gearbox"
  Generic_Engine_to_Central_Differential/1(Generic_Engine_to_Central_Differential) -> BCInputs/20  "Generic_Engine_to_Central_Differential"
  Generic_Engine_to_Front_Differential/1(Generic_Engine_to_Front_Differential) -> BCInputs/21  "Generic_Engine_to_Front_Differential"
  Generic_Engine_to_Rear_Differential/1(Generic_Engine_to_Rear_Differential) -> BCInputs/22  "Generic_Engine_to_Rear_Differential"
  Generic_Engine_to_Front_Right_Wheel/1(Generic_Engine_to_Front_Right_Wheel) -> BCInputs/23  "Generic_Engine_to_Front_Right_Wheel"
  Generic_Engine_to_Front_Left_Wheel/1(Generic_Engine_to_Front_Left_Wheel) -> BCInputs/24  "Generic_Engine_to_Front_Left_Wheel"
  Generic_Engine_to_Rear_Right_Wheel/1(Generic_Engine_to_Rear_Right_Wheel) -> BCInputs/25  "Generic_Engine_to_Rear_Right_Wheel"
  Generic_Engine_to_Rear_Left_Wheel/1(Generic_Engine_to_Rear_Left_Wheel) -> BCInputs/26  "Generic_Engine_to_Rear_Left_Wheel"
  Antiroll_Bar/1(Antiroll_Bar) -> BCInputs/27  "Antiroll_Bar"
  Aerodynamic/1(Aerodynamic) -> BCInputs/28  "Aerodynamic"
  Irregularity/1(Irregularity) -> BCInputs/29  "Irregularity"
  Main_Damper/1(Main_Damper) -> BCInputs/30  "Main_Damper"
  Main_Spring/1(Main_Spring) -> BCInputs/31  "Main_Spring"
  Main_Bumpstop/1(Main_Bumpstop) -> BCInputs/32  "Main_Bumpstop"
  Main_Reboundstop/1(Main_Reboundstop) -> BCInputs/33  "Main_Reboundstop"
  Auxiliary_vertical/1(Auxiliary_vertical) -> BCInputs/34  "Auxiliary_vertical"
  Main_Inerter/1(Main_Inerter) -> BCInputs/35  "Main_Inerter"
  Third_Element/1(Third_Element) -> BCInputs/36  "Third_Element"
  Mono_Element/1(Mono_Element) -> BCInputs/37  "Mono_Element"
  Tire_Force/1(Tire_Force) -> BCInputs/38  "Tire_Force"
  Tire_Moment/1(Tire_Moment) -> BCInputs/39  "Tire_Moment"
  Wheel_driving/1(Wheel_driving) -> BCInputs/40  "Wheel_driving"
  Ext_Body/1(Ext_Body) -> BCInputs/41  "Ext_Body"
  Ext_Ground/1(Ext_Ground) -> BCInputs/42  "Ext_Ground"
  Ext_Tracking/1(Ext_Tracking) -> BCInputs/43  "Ext_Tracking"
